simulink model "figure1"  (R2022a)
settings: Solver=FixedStepAuto  StartTime=0.0  StopTime=20  FixedStep=1  RelTol=1e-3
settings Model: Creator=SoLoMoN  LastModifiedBy=SoLoMoN

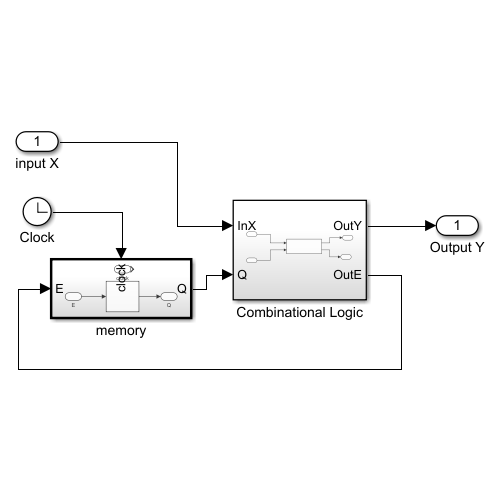
[thumbnail: Simulink's stored preview of the top-level diagram]
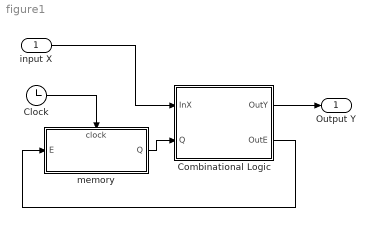
== system figure1 ==
  input X : Inport
  Clock : Clock
  Combinational Logic : Subsystem
  memory : Subsystem  TreatAsAtomicUnit=on
      settings: PortSchema="{\"entries\":[{\"content\":{\"sides\":[{\"content\":{\"connectorIds\":[\"In1\"]},\"type\":\"ConnectorPlacement.EquallySpacedRectSide\",\"uuid\":\"77aadec3-40b4-4159-965a-901ce092cc10\"},{\"content\":{\"connectorIds\":[\"Out1\"],\"side\":\"RIGHT\"},\"type\":\"ConnectorPlacement.EquallySpacedRectSide\",\"uuid\":\"7767cfc0-df44-4395-aad0-907ec8a11636\"},{\"content\":{\"connectorIds\":[\"In2\"],\"side\":\"TOP\"},\"type\":\"ConnectorPlacement.EquallySpacedRectSide\",\"uuid\":\"e3bba812-e96d-4ad6-88e6-3ed29f8a8dca\"}]},\"type\":\"ConnectorPlacement.EquallySpacedConnector\",\"uuid\":\"f3f8c250-2af8-41a3-af49-c856e11dc8d6\"}],\"packageUris\":[\"http://schema.mathworks.com/mf0/Connector/R2020b\"],\"version\":\"1.0\"}"
  Output Y : Outport
  wires:
  memory/1(Q) -> Combinational Logic/2(Q)
  Combinational Logic/1(OutY) -> Output Y/1
  Clock/1 -> memory/2(clock)
  input X/1 -> Combinational Logic/1(InX)
  Combinational Logic/2(OutE) -> memory/1(E)

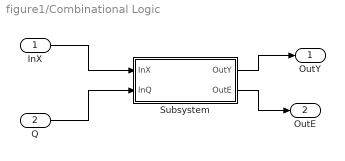
== system figure1/Combinational Logic ==
  InX : Inport
  Q : Inport  Port=2
  Subsystem : Subsystem
  OutY : Outport
  OutE : Outport  Port=2
  wires:
  InX/1 -> Subsystem/1(InX)
  Q/1 -> Subsystem/2(InQ)
  Subsystem/1(OutY) -> OutY/1
  Subsystem/2(OutE) -> OutE/1

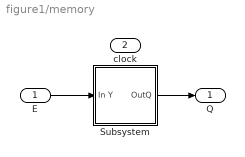
== system figure1/memory ==
  E : Inport
  clock : Inport  Port=2
  Subsystem : Subsystem
  Q : Outport
  wires:
  E/1 -> Subsystem/1(In Y)
  Subsystem/1(OutQ) -> Q/1

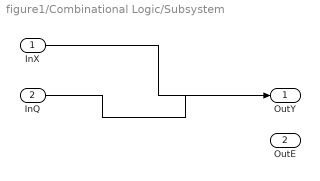
== system figure1/Combinational Logic/Subsystem ==
  InX : Inport
  InQ : Inport  Port=2
  OutY : Outport
  OutE : Outport  Port=2
  wires:
  InX/1 -> OutY/1
  InQ/1 -> ?

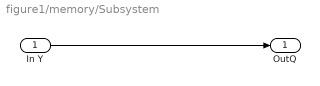
== system figure1/memory/Subsystem ==
  In Y : Inport
  OutQ : Outport
  wires:
  In Y/1 -> OutQ/1
